simulink model "hitCrossing1"  (R2017b)
settings: Solver=FixedStepAuto  StartTime=0.0  StopTime=10.0  FixedStep=1.000000  RelTol=1e-3
settings Model: Creator=hbourbou  LastModifiedBy=hbourbou

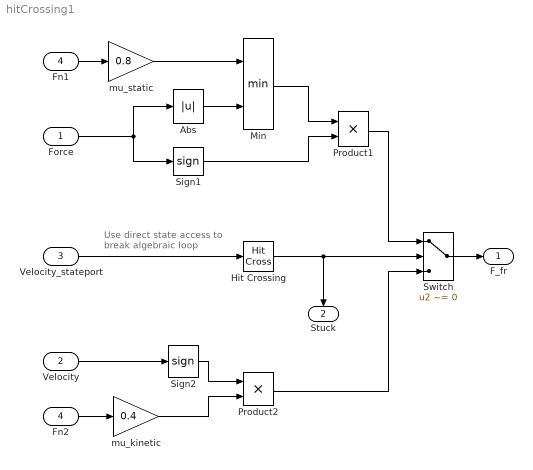
== system hitCrossing1 ==
  note: Use direct state access to
      | break algebraic loop
  Force : Inport
  Velocity : Inport  Port=2
  Velocity_stateport : Inport  Port=3
  Fn2 : Inport  Port=4
  Abs : Abs  SaturateOnIntegerOverflow=on
  Fn1 : InportShadow  Port=4
  Hit Crossing : HitCross
  Min : MinMax  Inputs=2  SaturateOnIntegerOverflow=on  InputSameDT=on
  Product1 : Product  SaturateOnIntegerOverflow=on  InputSameDT=on  OutDataTypeStr=Inherit: Same as first input
  Product2 : Product  SaturateOnIntegerOverflow=on  InputSameDT=on  OutDataTypeStr=Inherit: Same as first input
  Sign1 : Signum
  Sign2 : Signum
  Switch : Switch  Criteria=u2 ~= 0  Threshold=0.5  InputSameDT=on
  mu_kinetic : Gain  Gain=0.4
  mu_static : Gain  Gain=0.8
  F_fr : Outport  InitialOutput=0
  Stuck : Outport  Port=2  InitialOutput=0
  wires:
  mu_static/1 -> Min/1
  Product2/1 -> Switch/3
  Abs/1 -> Min/2
  Force/1 -> Abs/1, Sign1/1
  Fn1/1 -> mu_static/1
  Min/1 -> Product1/1
  Velocity/1 -> Sign2/1
  Sign2/1 -> Product2/1
  Switch/1 -> F_fr/1
  Velocity_stateport/1 -> Hit Crossing/1
  Sign1/1 -> Product1/2
  Product1/1 -> Switch/1
  Fn2/1 -> mu_kinetic/1
  mu_kinetic/1 -> Product2/2
  Hit Crossing/1 -> Stuck/1, Switch/2
